simulink model "lab3CTSys2_NEW"  (Simulink 7.1)
settings: Solver=ode45  SolverMode=SingleTasking  StartTime=0.0  StopTime=10  MaxStep=.05  RelTol=1e-3  AbsTol=1e-6
settings Model: Creator=vise  LastModifiedBy=vise  ExtModeTrigMode=oneshot  ExtModeArmWhenConnect=off  ExtModeAutoUpdateStatusClock=off
settings DataIOCC: LimitDataPoints=off
settings OptimizationCC: BooleanDataType=off
settings DebuggingCC: SaveWithParameterizedLinksMsg=none  SignalResolutionControl=TryResolveAllWithWarning  SolverPrmCheckMsg=none  MultiTaskDSMMsg=warning  MultiTaskCondExecSysMsg=none  StrictBusMsg=None
settings HardwareCC: TargetUnknown=on
settings RTWCC: TemplateMakefile=grt_unix.tmf  IncludeERTFirstTime=on

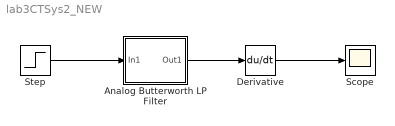
== system lab3CTSys2_NEW ==
  Analog Butterworth LP Filter : Subsystem  mask(buttap){@1=2*pi, @2=4}
      mask prompts: @1 "Cutoff frequency (rad/sec)"; @2 "Order"
      mask help:
      | Analog Butterworth low pass filter.
      |
      | (Requires Signal Processing Toolbox)
      mask init:
      | [z,p,k]=buttap(@2); z=@1*z; p=@1*p; k=real(prod(-p)); [num,den]=zp2tf(z,p,k); w=logspace(log10(@1/10),log10(10*@1),20); h=freqs(num,den,w);
      mask Help: Butterworth low pass filter using MATLAB's butter command.
      mask Display: plot(20*log10(w),20*log10(abs(h)))
  Derivative : Derivative
  Scope : Scope
      settings: TickLabels=on  DataFormat=Array
  Step : Step  Time=0.00001  SampleTime=0
  wires:
  Analog Butterworth LP Filter/1(Out1) -> Derivative/1
  Step/1 -> Analog Butterworth LP Filter/1(In1)
  Derivative/1 -> Scope/1

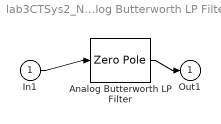
== system lab3CTSys2_NEW/Analog Butterworth LP Filter ==
  In1 : Inport
  Analog Butterworth LP Filter : ZeroPole  Zeros=z  Poles=p  Gain=k
  Out1 : Outport
  wires:
  In1/1 -> Analog Butterworth LP Filter/1
  Analog Butterworth LP Filter/1 -> Out1/1
